simulink model "TBRe18_ECU_V7_AI"  (R2017b)
settings: Solver=FixedStepDiscrete  StartTime=0.0  StopTime=inf  FixedStep=0.0001  RelTol=1e-3
PostLoadFcn:
  | model_init();
libraries: simulink x16, simulink_extras x1
(part 4 of 4)

== system TBRe18_ECU_V7_AI/Data_Processing/Diagnostics/ECU_I//0s_Diagnostics/LV_Battery ==
  In1 : Inport
  Bus Creator : BusCreator  Inputs=3
  Bus Selector : BusSelector  OutputSignals=LV_Battery_Voltage
  Data Type Conversion : DataTypeConversion  OutDataTypeStr=uint8
  LV_Warning_% : simulink/Logic and Bit Operations/Compare To Constant  relop=<=  const=20  OutDataTypeStr=boolean
  Voltage_Act : Lookup_n-D  NumberOfTableDimensions=1  BreakpointsForDimension1=[0,20000]  Table=[500,33000]  TableDataTypeStr=Inherit: Inherit from 'Table data'  ExtrapMethod=Clip  UseLastTableValue=on  InternalRulePriority=Speed  RndMeth=Simplest  InputSameDT=on
  "Voltage_SOC " : Lookup_n-D  NumberOfTableDimensions=1  BreakpointsForDimension1=[1600, 24000, 25800, 26000, 26400]  Table=[0, 10, 20, 50, 100]  TableDataTypeStr=Inherit: Inherit from 'Table data'  ExtrapMethod=Clip  UseLastTableValue=on  InternalRulePriority=Speed  RndMeth=Simplest  InputSameDT=on
  Out1 : Outport
  wires:
  Bus Creator/1 -> Out1/1
  In1/1 -> Bus Selector/1
  LV_Warning_%/1 -> Bus Creator/1  "LV_Battery_Warning"
  "Voltage_SOC "/1 -> Data Type Conversion/1, LV_Warning_%/1
  Data Type Conversion/1 -> Bus Creator/2  "LV_Battery_SOC"
  Bus Selector/1 -> Voltage_Act/1, "Voltage_SOC "/1  "<LV_Battery_Voltage>"
  Voltage_Act/1 -> Bus Creator/3  "LV_Battery_Voltage"

== system TBRe18_ECU_V7_AI/Data_Processing/Diagnostics/ECU_I//0s_Diagnostics/Pedal_Box ==
  In1 : Inport
  APPS and BP Plausibility : MATLAB Function  TreatAsAtomicUnit=on
  APPS_Implausibility_Check : MATLAB Function  TreatAsAtomicUnit=on
  Bus Creator : BusCreator  Inputs=10
  Bus Selector : BusSelector  OutputSignals=Pedal_Box_Data.Throttle1_Voltage,Pedal_Box_Data.Throttle2_Voltage,Pedal_Box_Data.Brake_Voltage
  Ground : Ground
  Sensor_Diag : MATLAB Function  TreatAsAtomicUnit=on
  Terminator : Terminator
  Voltage_to_% Conversion : Subsystem
  prv_BSPD : Delay  DelayLength=1  InitialCondition=0
  Out1 : Outport
  wires:
  Bus Creator/1 -> Out1/1
  In1/1 -> Bus Selector/1
  Bus Selector/1 -> Sensor_Diag/1(TV_1), Bus Creator/1  "<Throttle1_Voltage>"
  Bus Selector/3 -> Sensor_Diag/3(BV_1), Bus Creator/3  "<Brake_Voltage>"
  APPS and BP Plausibility/2(APPS_BP_Implausibility) -> prv_BSPD/1, Bus Creator/10  "APPS_BP_Implausibility"
  APPS and BP Plausibility/1(Throttle_Percentage) -> Bus Creator/9  "Throttle_%"
  Sensor_Diag/1(Pedal_Sensor_Fail) -> APPS_Implausibility_Check/1(Pedal_Sensor_Fail), Bus Creator/4  "Pedal_Sensor_Fail"
  APPS_Implausibility_Check/1(APPS_Implausbility) -> Bus Creator/8  "APPS_Implausibility"
  APPS_Implausibility_Check/2(Throttle_Percentage) -> Terminator/1
  Voltage_to_% Conversion/3(Out3) -> APPS and BP Plausibility/2(Brake_In), Bus Creator/7
  Sensor_Diag/2(TV1_Out) -> Voltage_to_% Conversion/1(In1)
  Sensor_Diag/3(TV2_Out) -> Voltage_to_% Conversion/2(In2)
  Sensor_Diag/4(BV_Out) -> Voltage_to_% Conversion/3(In3)
  Voltage_to_% Conversion/1(Out1) -> APPS and BP Plausibility/1(Throttle_In), Bus Creator/5
  Bus Selector/2 -> Sensor_Diag/2(TV_2), Bus Creator/2  "<Throttle2_Voltage>"
  Voltage_to_% Conversion/2(Out2) -> Bus Creator/6, APPS_Implausibility_Check/3(Throttle2_Per)
  prv_BSPD/1 -> APPS and BP Plausibility/3(APPS_BP_Implausibility_Prv)
  Ground/1 -> APPS_Implausibility_Check/2(Throttle1_Per)

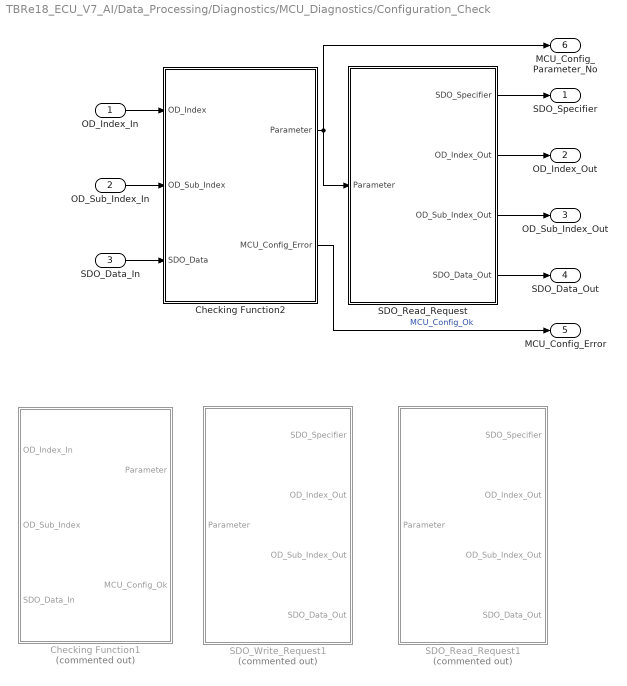
== system TBRe18_ECU_V7_AI/Data_Processing/Diagnostics/MCU_Diagnostics/Configuration_Check ==
  OD_Index_In : Inport
  OD_Sub_Index_In : Inport  Port=2
  SDO_Data_In : Inport  Port=3
  Checking Function1 : MATLAB Function  Commented=on  TreatAsAtomicUnit=on
  Checking Function2 : MATLAB Function  TreatAsAtomicUnit=on
  SDO_Read_Request : MATLAB Function  TreatAsAtomicUnit=on
  SDO_Read_Request1 : MATLAB Function  Commented=on  TreatAsAtomicUnit=on
  SDO_Write_Request1 : MATLAB Function  Commented=on  TreatAsAtomicUnit=on
  SDO_Specifier : Outport
  OD_Index_Out : Outport  Port=2
  OD_Sub_Index_Out : Outport  Port=3
  SDO_Data_Out : Outport  Port=4
  MCU_Config_Error : Outport  Port=5
  MCU_Config_Parameter_No : Outport  Port=6
  wires:
  Checking Function2/2(MCU_Config_Error) -> MCU_Config_Error/1  "MCU_Config_Ok"
  Checking Function2/1(Parameter) -> SDO_Read_Request/1(Parameter), MCU_Config_Parameter_No/1
  OD_Index_In/1 -> Checking Function2/1(OD_Index)
  SDO_Read_Request/3(OD_Sub_Index_Out) -> OD_Sub_Index_Out/1
  SDO_Data_In/1 -> Checking Function2/3(SDO_Data)
  SDO_Read_Request/1(SDO_Specifier) -> SDO_Specifier/1
  OD_Sub_Index_In/1 -> Checking Function2/2(OD_Sub_Index)
  SDO_Read_Request/4(SDO_Data_Out) -> SDO_Data_Out/1
  SDO_Read_Request/2(OD_Index_Out) -> OD_Index_Out/1

== system TBRe18_ECU_V7_AI/Data_Processing/Diagnostics/MCU_Diagnostics/Power Monitoring ==
  MCU_Input_Power : Inport
  Voltage_In : Inport  Port=2
  Current_In : Inport  Port=3
  Compare To Constant : simulink/Logic and Bit Operations/Compare To Constant  relop=>=  const=80000  OutDataTypeStr=boolean
  Gain : Gain  Gain=1000
  MinMax : MinMax  Function=max  Inputs=2
  Product : Product
  MCU_Power : Outport
  DC_Link_Voltage : Outport  Port=2
  DC_Link_Current : Outport  Port=3
  Power_Limit_Breach : Outport  Port=4
  wires:
  MinMax/1 -> Compare To Constant/1
  Voltage_In/1 -> Product/1, DC_Link_Voltage/1
  Current_In/1 -> Product/2, DC_Link_Current/1
  Product/1 -> MinMax/2
  Compare To Constant/1 -> Power_Limit_Breach/1
  MCU_Input_Power/1 -> Gain/1, MCU_Power/1
  Gain/1 -> MinMax/1

== system TBRe18_ECU_V7_AI/Data_Processing/Diagnostics/MCU_Diagnostics/Temp_Check ==
  MCU_Temp : Inport
  Motor_Temp : Inport  Port=2
  Max_Temp : simulink/Logic and Bit Operations/Compare To Constant  relop=>=  const=50  OutDataTypeStr=boolean
  MinMax : MinMax  Function=max  Inputs=2
  Pump_Start_Temp : simulink/Logic and Bit Operations/Compare To Constant  relop=>=  const=30  OutDataTypeStr=boolean
  MCU_Temperature : Outport
  Motor_Temperature : Outport  Port=2
  MCU_Motor_Temp_Error : Outport  Port=3
  MCU_Pump_Req : Outport  Port=4
  wires:
  MCU_Temp/1 -> MinMax/1, MCU_Temperature/1  "MCU_Temp"
  Motor_Temp/1 -> Motor_Temperature/1, MinMax/2  "Motor_Temp"
  MinMax/1 -> Pump_Start_Temp/1, Max_Temp/1
  Max_Temp/1 -> MCU_Motor_Temp_Error/1  "MCU_Motor_Temp_Error"
  Pump_Start_Temp/1 -> MCU_Pump_Req/1

== system TBRe18_ECU_V7_AI/Data_Processing/Vehicle_Functionality/Hardwired_Output_Functions/BSPD ==
  In1 : Inport
  In3 : Inport  Port=2
  Compare To Constant1 : simulink/Logic and Bit Operations/Compare To Constant  relop=>=  const=2500  OutDataTypeStr=boolean
  Compare To Constant2 : simulink/Logic and Bit Operations/Compare To Constant  relop=>=  const=2500  OutDataTypeStr=boolean
  Ground : Ground
  Logical Operator : Logic  AllPortsSameDT=off  OutDataTypeStr=boolean
  S-R Flip-Flop : simulink_extras/Flip Flops/S-R Flip-Flop  initial_condition=0
  Terminator : Terminator
  Out1 : Outport
  wires:
  Compare To Constant1/1 -> Logical Operator/1
  Compare To Constant2/1 -> Logical Operator/2
  Logical Operator/1 -> S-R Flip-Flop/1
  S-R Flip-Flop/1 -> Out1/1
  In1/1 -> Compare To Constant1/1
  In3/1 -> Compare To Constant2/1
  Ground/1 -> S-R Flip-Flop/2
  S-R Flip-Flop/2 -> Terminator/1

== system TBRe18_ECU_V7_AI/Data_Processing/Vehicle_Functionality/Vehicle_Operation_Mode/System_Error ==
  note: Shutdown Sig Not Working, BSPD dissconected
  In : Inport
  Bus Selector1 : BusSelector  OutputSignals=Shutdown_Data.Shutdown_Error,ECU_IO_Data.Pedal_Box_Data.APPS_BP_Implausibility,ECU_IO_Data.Pedal_Box_Data.APPS_Implausibility
  Ground : Ground
  Ground1 : Ground
  Ground2 : Ground
  Logical Operator : Logic  Operator=OR  Inputs=4  AllPortsSameDT=off  OutDataTypeStr=boolean
  Terminator : Terminator
  Terminator1 : Terminator
  Out : Outport
  wires:
  In/1 -> Bus Selector1/1  "Input_Data"
  Logical Operator/1 -> Out/1  "System_Error"
  Bus Selector1/1 -> Terminator/1  "<Shutdown_Error>"
  Bus Selector1/2 -> Terminator1/1  "<APPS_BP_Implausibility>"
  Bus Selector1/3 -> Logical Operator/4  "<APPS_Implausibility>"
  Ground/1 -> Logical Operator/1
  Ground1/1 -> Logical Operator/2
  Ground2/1 -> Logical Operator/3

== system TBRe18_ECU_V7_AI/Data_Processing/Diagnostics/ECU_I//0s_Diagnostics/Pedal_Box/Voltage_to_% Conversion ==
  In1 : Inport
  In2 : Inport  Port=2
  In3 : Inport  Port=3
  Data Type Conversion : DataTypeConversion  OutDataTypeStr=uint8
  Data Type Conversion1 : DataTypeConversion  OutDataTypeStr=uint8
  Data Type Conversion2 : DataTypeConversion  OutDataTypeStr=uint8
  Map1 : Lookup_n-D  NumberOfTableDimensions=1  BreakpointsForDimension1=[5170,6500]  Table=[0,100]  ExtrapMethod=Clip  UseLastTableValue=on  InternalRulePriority=Speed  RndMeth=Simplest  InputSameDT=on
  Map2 : Lookup_n-D  NumberOfTableDimensions=1  BreakpointsForDimension1=[6500,8000]  Table=[0,100]  ExtrapMethod=Clip  UseLastTableValue=on  InternalRulePriority=Speed  RndMeth=Simplest  InputSameDT=on
  Map3 : Lookup_n-D  NumberOfTableDimensions=1  BreakpointsForDimension1=[1300,5600]  Table=[0,100]  ExtrapMethod=Clip  UseLastTableValue=on  InternalRulePriority=Speed  RndMeth=Simplest  InputSameDT=on
  Out1 : Outport
  Out2 : Outport  Port=2
  Out3 : Outport  Port=3
  wires:
  Data Type Conversion/1 -> Out3/1  "Brake_%"
  In3/1 -> Map3/1
  In1/1 -> Map1/1
  In2/1 -> Map2/1
  Map3/1 -> Data Type Conversion/1
  Data Type Conversion1/1 -> Out1/1  "Throttle1_%"
  Map1/1 -> Data Type Conversion1/1
  Data Type Conversion2/1 -> Out2/1  "Throttle2_%"
  Map2/1 -> Data Type Conversion2/1

== matlab function TBRe18_ECU_V7_AI/Data_Processing/Vehicle_Functionality/Vehicle_Operation_Mode/Vehical Mode Selection ==
  data: Throttle input; Brake input; Reset input; Push_to_Start input; Error input; Prev_Operation_Mode input; MCU_NMT_Mode output; PWM output; Operation_Mode output; Buzzer output; Buzzer_Timer_In input; Buzzer_Timer_Out output; Precharge_Hold input
function [ MCU_NMT_Mode, PWM, Operation_Mode, Buzzer, Buzzer_Timer_Out] = Vehicle_Operation_Mode(Throttle, Brake,Reset, Push_to_Start,Error, Prev_Operation_Mode, Buzzer_Timer_In, Precharge_Hold)

%Parameter Initialisation
PWM = false;
Buzzer = false;
Buzzer_Timer_Out = 0;
Operation_Mode = Prev_Operation_Mode;

%Error checker
if (Error)
    Operation_Mode = uint8(0);
    MCU_NMT_Mode = uint8(0); %Stopped
end

%% -------------Vehicle Operation Modes--------------------%%

switch Operation_Mode
    
    case 0 %Error_Mode/No_Mode
        PWM = false;
        MCU_NMT_Mode = uint8(0); %Stopped Mode
        
        if (~Error)
            Operation_Mode = uint8(1);
        end
        
    case 1 %Standby_Mode: When car is first turned on
        PWM = false;
        MCU_NMT_Mode = uint8(2); %Pre-Operational Mode
        if (Brake && Push_to_Start && ~Throttle && (Precharge_Hold == 1))
            Operation_Mode = uint8(2);
            Buzzer_Timer_Out = 15;
        else
            Operation_Mode = uint8(1);
        end
        
    case 2 %Ready_to_Drive_Buzzer_Mode: Buzzer sounds before drive
        Buzzer = true;
        MCU_NMT_Mode = uint8(2); %Pre-Operational Mode
        if (Buzzer_Timer_In == 0)
            Buzzer = false;
            Operation_Mode = uint8(3);
        else
        Buzzer_Timer_Out = Buzzer_Timer_In - 1;
        Operation_Mode = uint8(2);
        end
        
    case 3 %Ready_to_Drive_Mode
        PWM = true;
        MCU_NMT_Mode = uint8(3); %Operational Mode
        if (Reset || (Precharge_Hold ~= 1))
            Operation_Mode = uint8(4);
        end
        
    case 4 %Reset Mode
        PWM = false;
        MCU_NMT_Mode = uint8(0); %Stopped Mode
        if (Reset)
            Operation_Mode = uint8(4); %Reset Mode
        else 
            Operation_Mode = uint8(0); %No Mode/Error Mode
        end
        
    otherwise 
        PWM = false;
        MCU_NMT_Mode = uint8(0);
        Operation_Mode = uint8(0);
end

end

== matlab function TBRe18_ECU_V7_AI/High_Priority_CAN_TX/MATLAB Function ==
  data: MCU_NMT_Mode input; Stopped output; Reset output; Pre_Op output; Op output
    function [Stopped,Reset,Pre_Op, Op]  = fcn(MCU_NMT_Mode)

Stopped = false;
Reset = false;
Pre_Op = false;
Op = false;

switch MCU_NMT_Mode
    case 0 %Stopped
        Stopped = true;
    case 1 %Reset
        Reset = true;
    case 2 %Pre-Op
        Pre_Op = true;
    case 3 %Op
        Op = true;
   
end

== matlab function TBRe18_ECU_V7_AI/Data_Processing/Diagnostics/BMS_Diagnostics/MATLAB Function ==
  data: Pack_Voltage input; Pre_Charge_Hold output; MCU_Link_Voltage input
function Pre_Charge_Hold = fcn(Pack_Voltage, MCU_Link_Voltage)
%Pre-Charge line hold
MCU_Link_Voltage = double(MCU_Link_Voltage);

Threshold = 0.90*Pack_Voltage;
%Added Check for voltage above 60V so precharge is not open when car turns
%on or no accumilator in car

if(((MCU_Link_Voltage/10) >= Threshold) && (MCU_Link_Voltage >= 60) && Pack_Voltage >= 200)
    Pre_Charge_Hold = true;
else
    Pre_Charge_Hold = false;
end

end

== matlab function TBRe18_ECU_V7_AI/Data_Processing/Diagnostics/MCU_Diagnostics/Configuration_Check/Checking Function1 ==
  data: Parameter output; OD_Index_In input; OD_Sub_Index input; SDO_Data_In input; MCU_Config_Ok output
function [Parameter, MCU_Config_Ok] = Checking(OD_Index_In,OD_Sub_Index, SDO_Data_In)
%Configuration parameter checking function
switch OD_Index_In
    case 0
        MCU_Config_Ok = false;
        Parameter = uint8(1);
        
    case 8244 %Motor type = 0 (PSM)
        MCU_Config_Ok = false;
        if (SDO_Data_In == 0)
            Parameter = uint8(2);
        else
            Parameter = uint8(1);
        end
        
    case 8249 %FOC_Delay = 1 (Enabled)
        if (SDO_Data_In == 1)
            MCU_Config_Ok = false;
            Parameter = uint8(3);
        else
            MCU_Config_Ok = false;
            Parameter = uint8(2);
        end
        
    case 8243 %Motor Pole Pairs = 10 Pole Pairs
        if (SDO_Data_In == 10)
            MCU_Config_Ok = false;
            Parameter = uint8(4);
        else
            MCU_Config_Ok = false;
            Parameter = uint8(3);
        end
        
    case 24693 %Motor Rated Current = 320A
        if (SDO_Data_In == 320000)
            MCU_Config_Ok = false;
            Parameter = uint8(5);
        else
            MCU_Config_Ok = false;
            Parameter = uint8(4);
        end
    case 24694 %Motor Rated Torque = 320Nm
        if (SDO_Data_In == 320000)
            MCU_Config_Ok = false;
            Parameter = uint8(6);
        else
            MCU_Config_Ok = false;
            Parameter = uint8(5);
        end
    case 8279 %Motor Temperature Sensor = 3 (kty 81/210)
        if (SDO_Data_In == 3)
            MCU_Config_Ok = false;
            Parameter = uint8(7);
        else
            MCU_Config_Ok = false;
            Parameter = uint8(6);
        end
        
        %%-----------FEEDBACK PARAMETERS-----------&&
    case 8256
        %Feedback Type
        if (SDO_Data_In == 2 && OD_Sub_Index == 1)
            MCU_Config_Ok = false;
            Parameter = uint8(8);
            
            %Feedback Resolution
        elseif (SDO_Data_In == 4096 && OD_Sub_Index == 6)
            MCU_Config_Ok = false;
            Parameter = uint8(9);
            
            %Auto aligning motor position current
        elseif (SDO_Data_In == 500 && OD_Sub_Index == 10)
            MCU_Config_Ok = false;
            Parameter = uint8(10);
            
            %Motor phase offset compensation
        elseif (SDO_Data_In == 190 && OD_Sub_Index == 8)
            MCU_Config_Ok = false;
            Parameter = uint8(11);
        else
            MCU_Config_Ok = false;
            Parameter = uint8(8);
        end
        
        %%-----------BATTERY PARAMETERS-----------&&
    case 8276 %Overvoltage limit = 400V
        if (SDO_Data_In == 400)
            MCU_Config_Ok = false;
            Parameter = uint8(12);
        else
            MCU_Config_Ok = false;
            Parameter = uint8(11);
        end
    case 8277
        %Undervoltage limit = 200V
        if (SDO_Data_In == 200 && OD_Sub_Index == 1)
            MCU_Config_Ok = false;
            Parameter = uint8(13);
            %Undervoltage limit gain = 20%/V
        elseif (SDO_Data_In == 20 && OD_Sub_Index == 2)
            MCU_Config_Ok = false;
            Parameter = uint8(14);
            %Undervoltage min voltage = 195V
        elseif (SDO_Data_In == 195 && OD_Sub_Index == 3)
            MCU_Config_Ok = false;
            Parameter = uint8(15);
        else
            MCU_Config_Ok = false;
            Parameter = uint8(12);
        end
        
    case 4112 %Parameter Save
        if (SDO_Data_In == 1702257011)
            MCU_Config_Ok = true;
            Parameter = uint8(0);
        else
            MCU_Config_Ok = false;
            Parameter = uint8(15);
        end
        
    otherwise
        MCU_Config_Ok = false;
        Parameter = uint8(1);
        
end
end

== matlab function TBRe18_ECU_V7_AI/Data_Processing/Diagnostics/MCU_Diagnostics/Configuration_Check/SDO_Write_Request1 ==
  data: Parameter input; SDO_Specifier output; OD_Index_Out output; OD_Sub_Index_Out output; SDO_Data_Out output
function [SDO_Specifier, OD_Index_Out, OD_Sub_Index_Out, SDO_Data_Out] = SDO_Write_Request(Parameter)
%Auto-align procedure parameter check

switch Parameter
    %%-----------MOTOR PARAMETERS-----------&&
    case 1 %Motor type
        SDO_Specifier = uint8(47); %Write
        OD_Index_Out = uint16(8244); %OD Index
        OD_Sub_Index_Out = uint8(0); %OD Sub-Index
        SDO_Data_Out = uint32(0); %SDO Data - specific value
    case 2 %FOC_Delay
        SDO_Specifier = uint8(47); %Write
        OD_Index_Out = uint16(8249); %OD Index
        OD_Sub_Index_Out = uint8(0); %OD Sub-Index
        SDO_Data_Out = uint32(1); %SDO Data - specific value
    case 3 %Motor Pole Pairs
        SDO_Specifier = uint8(47); %Write
        OD_Index_Out = uint16(8243); %OD Index
        OD_Sub_Index_Out = uint8(0); %OD Sub-Index
        SDO_Data_Out = uint32(10); %SDO Data - specific value
    case 4 %Motor Rated Current
        SDO_Specifier = uint8(47); %Write
        OD_Index_Out = uint16(24693); %OD Index
        OD_Sub_Index_Out = uint8(0); %OD Sub-Index
        SDO_Data_Out = uint32(320000); %SDO Data - specific value
    case 5 %Motor Rated Torque
        SDO_Specifier = uint8(47); %Write
        OD_Index_Out = uint16(24694); %OD Index
        OD_Sub_Index_Out = uint8(0); %OD Sub-Index
        SDO_Data_Out = uint32(320000); %SDO Data - specific value
    case 6 %Motor Temperature Sensor
        SDO_Specifier = uint8(47); %Write
        OD_Index_Out = uint16(8279); %OD Index
        OD_Sub_Index_Out = uint8(2); %OD Sub-Index
        SDO_Data_Out = uint32(3); %SDO Data - specific value
        
       %%-----------FEEDBACK PARAMETERS-----------&&
    case 7 %Feedback Type
        SDO_Specifier = uint8(47); %Write
        OD_Index_Out = uint16(8256); %OD Index
        OD_Sub_Index_Out = uint8(1); %OD Sub-Index
        SDO_Data_Out = uint32(2); %SDO Data - specific value
    case 8 %Feedback Resolution
        SDO_Specifier = uint8(47); %Write
        OD_Index_Out = uint16(8256); %OD Index
        OD_Sub_Index_Out = uint8(6); %OD Sub-Index
        SDO_Data_Out = uint32(4096); %SDO Data - specific value
    case 9 %Auto aligning motor position current
        SDO_Specifier = uint8(47); %Write
        OD_Index_Out = uint16(8256); %OD Index
        OD_Sub_Index_Out = uint8(10); %OD Sub-Index
        SDO_Data_Out = uint32(500); %SDO Data - specific value
    case 10 %Motor phase offset compensation
        SDO_Specifier = uint8(47); %Write
        OD_Index_Out = uint16(8256); %OD Index
        OD_Sub_Index_Out = uint8(8); %OD Sub-Index
        SDO_Data_Out = uint32(190); %SDO Data - specific value
        
        %%-----------BATTERY PARAMETERS-----------&&
    case 11 %Overvoltage limit
        SDO_Specifier = uint8(47); %Write
        OD_Index_Out = uint16(8276); %OD Index
        OD_Sub_Index_Out = uint8(1); %OD Sub-Index
        SDO_Data_Out = uint32(400); %SDO Data - specific value
    case 12 %Undervoltage limit
        SDO_Specifier = uint8(47); %Write
        OD_Index_Out = uint16(8277); %OD Index
        OD_Sub_Index_Out = uint8(1); %OD Sub-Index
        SDO_Data_Out = uint32(200); %SDO Data - specific value
    case 13 %Undervoltage limit gain
        SDO_Specifier = uint8(47); %Write
        OD_Index_Out = uint16(8277); %OD Index
        OD_Sub_Index_Out = uint8(2); %OD Sub-Index
        SDO_Data_Out = uint32(20); %SDO Data - specific value
    case 14 %Undervoltage min voltage
        SDO_Specifier = uint8(47); %Write
        OD_Index_Out = uint16(8277); %OD Index
        OD_Sub_Index_Out = uint8(3); %OD Sub-Index
        SDO_Data_Out = uint32(195); %SDO Data - specific value
    case 15 %Parameter Save
        SDO_Specifier = uint8(47); %Write
        OD_Index_Out = uint16(4112); %OD Index
        OD_Sub_Index_Out = uint8(1); %OD Sub-Index
        SDO_Data_Out = uint32(1702257011); %SDO Data - specific value
    otherwise
        SDO_Specifier = uint8(0); %Read
        OD_Index_Out = uint16(0); %OD Index
        OD_Sub_Index_Out = uint8(0); %OD Sub-Index
        SDO_Data_Out = uint32(0); %SDO Data - specific value
end

end

== matlab function TBRe18_ECU_V7_AI/Data_Processing/Diagnostics/MCU_Diagnostics/Configuration_Check/SDO_Read_Request ==
  data: Parameter input; SDO_Specifier output; OD_Index_Out output; OD_Sub_Index_Out output; SDO_Data_Out output
function [SDO_Specifier, OD_Index_Out, OD_Sub_Index_Out, SDO_Data_Out] = SDO_Read_Request(Parameter)
%Configuration procedure parameter check

switch Parameter
    %%-----------MOTOR PARAMETERS-----------&&
    case 1 %Motor type
        SDO_Specifier = uint8(64); %Read Request
        OD_Index_Out = uint16(8244); %OD Index
        OD_Sub_Index_Out = uint8(0); %OD Sub-Index
        SDO_Data_Out = uint32(0); %SDO Data - specific value
    case 2 %FOC_Delay
        SDO_Specifier = uint8(64); %Read Request
        OD_Index_Out = uint16(8249); %OD Index
        OD_Sub_Index_Out = uint8(0); %OD Sub-Index
        SDO_Data_Out = uint32(0); %SDO Data - specific value
    case 3 %Motor Pole Pairs
        SDO_Specifier = uint8(64); %Read Request
        OD_Index_Out = uint16(8243); %OD Index
        OD_Sub_Index_Out = uint8(0); %OD Sub-Index
        SDO_Data_Out = uint32(0); %SDO Data - specific value
    case 4 %Motor Rated Current
        SDO_Specifier = uint8(64); %Read Request
        OD_Index_Out = uint16(24693); %OD Index
        OD_Sub_Index_Out = uint8(0); %OD Sub-Index
        SDO_Data_Out = uint32(0); %SDO Data - specific value
    case 5 %Motor Rated Torque
        SDO_Specifier = uint8(64); %Read Request
        OD_Index_Out = uint16(24694); %OD Index
        OD_Sub_Index_Out = uint8(0); %OD Sub-Index
        SDO_Data_Out = uint32(0); %SDO Data - specific value
    case 6 %Motor Temperature Sensor
        SDO_Specifier = uint8(64); %Read Request
        OD_Index_Out = uint16(8279); %OD Index
        OD_Sub_Index_Out = uint8(1); %OD Sub-Index
        SDO_Data_Out = uint32(0); %SDO Data - specific value
        
       %%-----------FEEDBACK PARAMETERS-----------%%
    case 7 %Feedback Type
        SDO_Specifier = uint8(64); %Read Request
        OD_Index_Out = uint16(8256); %OD Index
        OD_Sub_Index_Out = uint8(1); %OD Sub-Index
        SDO_Data_Out = uint32(0); %SDO Data - specific value
    case 8 %Feedback Resolution
        SDO_Specifier = uint8(64); %Read Request
        OD_Index_Out = uint16(8256); %OD Index
        OD_Sub_Index_Out = uint8(6); %OD Sub-Index
        SDO_Data_Out = uint32(0); %SDO Data - specific value
    case 9 %Auto aligning motor position current
        SDO_Specifier = uint8(64); %Read Request
        OD_Index_Out = uint16(8256); %OD Index
        OD_Sub_Index_Out = uint8(10); %OD Sub-Index
        SDO_Data_Out = uint32(0); %SDO Data - specific value
    case 10 %Motor phase offset compensation
        SDO_Specifier = uint8(64); %Read Request
        OD_Index_Out = uint16(8256); %OD Index
        OD_Sub_Index_Out = uint8(8); %OD Sub-Index
        SDO_Data_Out = uint32(0); %SDO Data - specific value
        
        %%-----------BATTERY PARAMETERS-----------&&
    case 11 %Overvoltage limit
        SDO_Specifier = uint8(64); %Read Request
        OD_Index_Out = uint16(8276); %OD Index
        OD_Sub_Index_Out = uint8(0); %OD Sub-Index
        SDO_Data_Out = uint32(0); %SDO Data - specific value
    case 12 %Undervoltage limit
        SDO_Specifier = uint8(64); %Read Request
        OD_Index_Out = uint16(8277); %OD Index
        OD_Sub_Index_Out = uint8(1); %OD Sub-Index
        SDO_Data_Out = uint32(0); %SDO Data - specific value
    case 13 %Undervoltage limit gain
        SDO_Specifier = uint8(64); %Read Request
        OD_Index_Out = uint16(8277); %OD Index
        OD_Sub_Index_Out = uint8(2); %OD Sub-Index
        SDO_Data_Out = uint32(0); %SDO Data - specific value
    case 14 %Undervoltage min voltage
        SDO_Specifier = uint8(64); %Read Request
        OD_Index_Out = uint16(8277); %OD Index
        OD_Sub_Index_Out = uint8(3); %OD Sub-Index
        SDO_Data_Out = uint32(0); %SDO Data - specific value
    case 15 %Parameter Save
        SDO_Specifier = uint8(35); %Save
        OD_Index_Out = uint16(4112); %OD Index
        OD_Sub_Index_Out = uint8(1); %OD Sub-Index
        SDO_Data_Out = uint32(1702257011); %SDO Data - specific value
    otherwise
        SDO_Specifier = uint8(0); %Read
        OD_Index_Out = uint16(0); %OD Index
        OD_Sub_Index_Out = uint8(0); %OD Sub-Index
        SDO_Data_Out = uint32(0); %SDO Data - specific value
end

end

== matlab function TBRe18_ECU_V7_AI/Data_Processing/Diagnostics/MCU_Diagnostics/Configuration_Check/Checking Function2 ==
  data: Parameter output; OD_Index input; OD_Sub_Index input; SDO_Data input; MCU_Config_Error output
function [Parameter, MCU_Config_Error] = Checking(OD_Index,OD_Sub_Index, SDO_Data)
%Configuration parameter checking function
switch OD_Index
    case 0
        MCU_Config_Error = true;
        Parameter = uint8(1);
        
    case 8244 %Motor type = 0 (PSM)
        MCU_Config_Error = true;
        if (SDO_Data == 0)
            Parameter = uint8(2);
        else
            Parameter = uint8(1);
        end
        
    case 8249 %FOC_Delay = 1 (Enabled)
        if (SDO_Data == 1)
            MCU_Config_Error = true;
            Parameter = uint8(3);
        else
            MCU_Config_Error = true;
            Parameter = uint8(2);
        end
        
    case 8243 %Motor Pole Pairs = 10 Pole Pairs
        if (SDO_Data == 10)
            MCU_Config_Error = true;
            Parameter = uint8(4);
        else
            MCU_Config_Error = true;
            Parameter = uint8(3);
        end
        
    case 24693 %Motor Rated Current = 320A
        if (SDO_Data == 320000)
            MCU_Config_Error = true;
            Parameter = uint8(5);
        else
            MCU_Config_Error = true;
            Parameter = uint8(4);
        end
    case 24694 %Motor Rated Torque = 320Nm
        if (SDO_Data == 320000)
            MCU_Config_Error = true;
            Parameter = uint8(6);
        else
            MCU_Config_Error = true;
            Parameter = uint8(5);
        end
    case 8279 %Motor Temperature Sensor = 3 (kty 81/210)
        if (SDO_Data == 3)
            MCU_Config_Error = true;
            Parameter = uint8(7);
        else
            MCU_Config_Error = true;
            Parameter = uint8(6);
        end
        
        %%-----------FEEDBACK PARAMETERS-----------&&
    case 8256
        %Feedback Type
        if (SDO_Data == 2 && OD_Sub_Index == 1)
            MCU_Config_Error = true;
            Parameter = uint8(8);
            
            %Feedback Resolution
        elseif (SDO_Data == 4096 && OD_Sub_Index == 6)
            MCU_Config_Error = true;
            Parameter = uint8(9);
            
            %Auto aligning motor position current
        elseif (SDO_Data == 500 && OD_Sub_Index == 10)
            MCU_Config_Error = true;
            Parameter = uint8(10);
            
            %Motor phase offset compensation
        elseif (SDO_Data == 190 && OD_Sub_Index == 8)
            MCU_Config_Error = true;
            Parameter = uint8(11);
        else
            MCU_Config_Error = true;
            Parameter = uint8(7);
        end
        
        %%-----------BATTERY PARAMETERS-----------&&
    case 8276 %Overvoltage limit = 400V
        if (SDO_Data == 400)
            MCU_Config_Error = true;
            Parameter = uint8(12);
        else
            MCU_Config_Error = true;
            Parameter = uint8(11);
        end
    case 8277
        %Undervoltage limit = 200V
        if (SDO_Data == 200 && OD_Sub_Index == 1)
            MCU_Config_Error = true;
            Parameter = uint8(13);
            %Undervoltage limit gain = 20%/V
        elseif (SDO_Data == 20 && OD_Sub_Index == 2)
            MCU_Config_Error = true;
            Parameter = uint8(14);
            %Undervoltage min voltage = 195V
        elseif (SDO_Data == 195 && OD_Sub_Index == 3)
            MCU_Config_Error = true;
            Parameter = uint8(15);
        else
            MCU_Config_Error = true;
            Parameter = uint8(12);
        end
    case 4112 %Save Parameter
        MCU_Config_Error = false;
        Parameter = uint8(0);
        
    otherwise
        MCU_Config_Error = true;
        Parameter = uint8(1);
        
end
end

== matlab function TBRe18_ECU_V7_AI/Data_Processing/Diagnostics/MCU_Diagnostics/Configuration_Check/SDO_Read_Request1 ==
  data: Parameter input; SDO_Specifier output; OD_Index_Out output; OD_Sub_Index_Out output; SDO_Data_Out output
function [SDO_Specifier, OD_Index_Out, OD_Sub_Index_Out, SDO_Data_Out] = SDO_Read_Request(Parameter)
%Auto-align procedure parameter check

switch Parameter
    %%-----------MOTOR PARAMETERS-----------&&
    case 1 %Motor type
        SDO_Specifier = uint8(64); %Read Request
        OD_Index_Out = uint16(8244); %OD Index
        OD_Sub_Index_Out = uint8(0); %OD Sub-Index
        SDO_Data_Out = uint32(0); %SDO Data - specific value
    case 2 %FOC_Delay
        SDO_Specifier = uint8(64); %Read Request
        OD_Index_Out = uint16(8249); %OD Index
        OD_Sub_Index_Out = uint8(0); %OD Sub-Index
        SDO_Data_Out = uint32(0); %SDO Data - specific value
    case 3 %Motor Pole Pairs
        SDO_Specifier = uint8(64); %Read Request
        OD_Index_Out = uint16(8243); %OD Index
        OD_Sub_Index_Out = uint8(0); %OD Sub-Index
        SDO_Data_Out = uint32(0); %SDO Data - specific value
    case 4 %Motor Rated Current
        SDO_Specifier = uint8(64); %Read Request
        OD_Index_Out = uint16(24693); %OD Index
        OD_Sub_Index_Out = uint8(0); %OD Sub-Index
        SDO_Data_Out = uint32(0); %SDO Data - specific value
    case 5 %Motor Rated Torque
        SDO_Specifier = uint8(64); %Read Request
        OD_Index_Out = uint16(24694); %OD Index
        OD_Sub_Index_Out = uint8(0); %OD Sub-Index
        SDO_Data_Out = uint32(0); %SDO Data - specific value
    case 6 %Motor Temperature Sensor
        SDO_Specifier = uint8(64); %Read Request
        OD_Index_Out = uint16(8279); %OD Index
        OD_Sub_Index_Out = uint8(1); %OD Sub-Index
        SDO_Data_Out = uint32(0); %SDO Data - specific value
        
       %%-----------FEEDBACK PARAMETERS-----------%%
    case 7 %Feedback Type
        SDO_Specifier = uint8(64); %Read Request
        OD_Index_Out = uint16(8256); %OD Index
        OD_Sub_Index_Out = uint8(1); %OD Sub-Index
        SDO_Data_Out = uint32(0); %SDO Data - specific value
    case 8 %Feedback Resolution
        SDO_Specifier = uint8(64); %Read Request
        OD_Index_Out = uint16(8256); %OD Index
        OD_Sub_Index_Out = uint8(6); %OD Sub-Index
        SDO_Data_Out = uint32(0); %SDO Data - specific value
    case 9 %Auto aligning motor position current
        SDO_Specifier = uint8(64); %Read Request
        OD_Index_Out = uint16(8256); %OD Index
        OD_Sub_Index_Out = uint8(10); %OD Sub-Index
        SDO_Data_Out = uint32(0); %SDO Data - specific value
    case 10 %Motor phase offset compensation
        SDO_Specifier = uint8(64); %Read Request
        OD_Index_Out = uint16(8256); %OD Index
        OD_Sub_Index_Out = uint8(8); %OD Sub-Index
        SDO_Data_Out = uint32(0); %SDO Data - specific value
        
        %%-----------BATTERY PARAMETERS-----------&&
    case 11 %Overvoltage limit
        SDO_Specifier = uint8(64); %Read Request
        OD_Index_Out = uint16(8276); %OD Index
        OD_Sub_Index_Out = uint8(0); %OD Sub-Index
        SDO_Data_Out = uint32(0); %SDO Data - specific value
    case 12 %Undervoltage limit
        SDO_Specifier = uint8(64); %Read Request
        OD_Index_Out = uint16(8277); %OD Index
        OD_Sub_Index_Out = uint8(1); %OD Sub-Index
        SDO_Data_Out = uint32(0); %SDO Data - specific value
    case 13 %Undervoltage limit gain
        SDO_Specifier = uint8(64); %Read Request
        OD_Index_Out = uint16(8277); %OD Index
        OD_Sub_Index_Out = uint8(2); %OD Sub-Index
        SDO_Data_Out = uint32(0); %SDO Data - specific value
    case 14 %Undervoltage min voltage
        SDO_Specifier = uint8(64); %Read Request
        OD_Index_Out = uint16(8277); %OD Index
        OD_Sub_Index_Out = uint8(3); %OD Sub-Index
        SDO_Data_Out = uint32(0); %SDO Data - specific value
    case 15 %Parameter Save
        SDO_Specifier = uint8(35); %Save
        OD_Index_Out = uint16(4112); %OD Index
        OD_Sub_Index_Out = uint8(1); %OD Sub-Index
        SDO_Data_Out = uint32(1702257011); %SDO Data - specific value
    otherwise
        SDO_Specifier = uint8(0); %Read
        OD_Index_Out = uint16(0); %OD Index
        OD_Sub_Index_Out = uint8(0); %OD Sub-Index
        SDO_Data_Out = uint32(0); %SDO Data - specific value
end

end

== matlab function TBRe18_ECU_V7_AI/Data_Processing/Diagnostics/ECU_I//0s_Diagnostics/Pedal_Box/Sensor_Diag ==
  data: TV_1 input; Pedal_Sensor_Fail output; TV_2 input; TV1_Out output; TV2_Out output; BV_1 input; BV_Out output
function [Pedal_Sensor_Fail,TV1_Out,TV2_Out,BV_Out ] = Sensor_Diagnostics(TV_1,TV_2,BV_1)
%Checks whether the throttle sensors are in their calibrated range

%Initialisation of throttle outputs, default low 
TV1_Out=uint16(0);
TV2_Out=uint16(0);
BV_Out=uint16(0);

if (TV_1>8000 || TV_1<4000) %if V1 out of normal range
    Pedal_Sensor_Fail = uint8(1);
    if (TV_2>10000 || TV_2<6000)
        Pedal_Sensor_Fail = uint8(3); %if both throttle sensors out of normal range
    end
    if (BV_1>17000 || BV_1<0)
        Pedal_Sensor_Fail = uint8(5); %if all sensors out of normal range
    end
    
elseif (TV_2>10000 || TV_2<6000) %if V2 out of normal range
    Pedal_Sensor_Fail = uint8(2);
    
elseif (BV_1>17000 || BV_1<0) %if brake out of normal range
    Pedal_Sensor_Fail = uint8(4);

else %if no error pass voltages to pedal checks
    Pedal_Sensor_Fail= uint8(0);
    TV1_Out=uint16(TV_1);
    TV2_Out=uint16(TV_2);
    BV_Out=uint16(BV_1);
end

== matlab function TBRe18_ECU_V7_AI/Data_Processing/Diagnostics/ECU_I//0s_Diagnostics/Pedal_Box/APPS_Implausibility_Check ==
  data: Pedal_Sensor_Fail input; APPS_Implausbility output; Throttle1_Per input; Throttle2_Per input; Throttle_Percentage output
function [APPS_Implausbility, Throttle_Percentage] = APPS_Implausibility_Check(Pedal_Sensor_Fail, Throttle1_Per, Throttle2_Per)
%Limit generation for comparison
Upper_Limit = Throttle1_Per+15;
Lower_Limit = Throttle1_Per-15;

%Passes one throttle if in range and no pedal sensor errors
if ((Lower_Limit <= Throttle2_Per) && (Throttle2_Per <= Upper_Limit)&& Pedal_Sensor_Fail == 0)
    Throttle_Percentage = uint8(min(Throttle1_Per, Throttle2_Per));
    APPS_Implausbility = false;
%All other conditions result in no throttle being applied
else 
    Throttle_Percentage = uint8(0);
    APPS_Implausbility = true;
end 

end

== matlab function TBRe18_ECU_V7_AI/Data_Processing/Diagnostics/ECU_I//0s_Diagnostics/Pedal_Box/APPS and BP Plausibility ==
  data: Throttle_In input; Throttle_Percentage output; Brake_In input; APPS_BP_Implausibility output; APPS_BP_Implausibility_Prv input
function [Throttle_Percentage, APPS_BP_Implausibility] = APPS_BP_Plausibility_Check(Throttle_In, Brake_In, APPS_BP_Implausibility_Prv)
%Plausibility check on both throttle and brake

%Implausible case: when both brake and throttle applied
if (Brake_In >=20 && Throttle_In > 25)
    APPS_BP_Implausibility = true;
    Throttle_Percentage =uint8(0);
    
%Implausible case: when brake lifted but throttle still not below 5%
elseif (APPS_BP_Implausibility_Prv && Throttle_In > 5)
    APPS_BP_Implausibility = true;
    Throttle_Percentage =uint8(0);
    
%Plausible case, throttle goes below 5%
elseif (APPS_BP_Implausibility_Prv && Throttle_In < 5)
    APPS_BP_Implausibility = false;
    Throttle_Percentage =uint8(Throttle_In);
    
%Plausible case, normal operation
else
    APPS_BP_Implausibility = false;
    Throttle_Percentage =uint8(Throttle_In);
end

== matlab function TBRe18_ECU_V7_AI/Data_Processing/Vehicle_Functionality/Vehicle_Operation_Mode/Vehcile Mode No Reset ==
  data: Throttle input; Brake input; Push_to_Start input; Pre_Charge_Hold input; DriverlessRTD input; Error input; Prev_Operation_Mode input; Timer_In input; MCU_NMT_Mode output; PWM output; Operation_Mode output; Buzzer output; Timer_Out output
function [ MCU_NMT_Mode, PWM, Operation_Mode, Buzzer, Timer_Out] = Vehicle_Operation_Mode(Throttle, Brake, Push_to_Start, Pre_Charge_Hold, DriverlessRTD, Error, Prev_Operation_Mode, Timer_In)

%Parameter Initialisation
PWM = false;
Buzzer = false;
Timer_Out = uint8(0);
Operation_Mode = Prev_Operation_Mode;

%Error checker
if (Error)
    Operation_Mode = uint8(0);
    MCU_NMT_Mode = uint8(0); %Stopped
end

%% -------------Vehicle Operation Modes--------------------%%

switch Operation_Mode
    
    case 0 %Error_Mode/No_Mode
        PWM = false;
        MCU_NMT_Mode = uint8(0); %Stopped Mode
        
        if (~Error)
            Operation_Mode = uint8(1);
        end
        
    case 1 %Standby_Mode: When car is first turned on
        PWM = false;
        MCU_NMT_Mode = uint8(2); %Pre-Operational Mode
        if ((Brake && Push_to_Start && ~Throttle && Pre_Charge_Hold)||(Brake && DriverlessRTD && ~Throttle && Pre_Charge_Hold))
            Operation_Mode = uint8(2);
            Timer_Out = uint8(30); %1.5s
        elseif (Push_to_Start)
            Operation_Mode = uint8(0);
        else
            Operation_Mode = uint8(1);
        end
        
    case 2 %Ready_to_Drive_Buzzer_Mode: Buzzer sounds before drive
        Buzzer = true;
        MCU_NMT_Mode = uint8(2); %Pre-Operational Mode
        if (Timer_In == uint8(0))
            Buzzer = false;
            Operation_Mode = uint8(3);
        else
            Timer_Out = Timer_In - uint8(1);
            Operation_Mode = uint8(2);
        end
        
    case 3 %Ready_to_Drive_Mode
        PWM = true;
        MCU_NMT_Mode = uint8(3); %Operational Mode
        
        if (Push_to_Start||~Pre_Charge_Hold||~DriverlessRTD)
            Operation_Mode = uint8(0);
        end
        
    otherwise
        PWM = false;
        MCU_NMT_Mode = uint8(0);
        Operation_Mode = uint8(0);
end

end

== stateflow chart TBRe18_ECU_V7_AI/Data_Processing/Vehicle_Functionality/Vehicle_Operation_Mode/Chart ==
  state Standby State:
    Buzzer = false;
    PWM = false;
    MCU_NMT_Mode = uint8(2); %Pre-Operational Mode
  state Error State:
    Buzzer = false;
    PWM = false;
    MCU_NMT_Mode = uint8(0); %Stopped Mode
  state Buzzer State:
    PWM = false;
    Buzzer = true;
    MCU_NMT_Mode = uint8(2); %Pre-Operational Mode
  state R2D State:
    Buzzer = false;
    PWM = true;
    MCU_NMT_Mode = uint8(3); %Operational Mode
  (default) -> Error State:
  Error State: -> Standby State: : [~Error]
  Standby State: -> Error State: [order 1] : [Error || (btnDash && ~Brake)]
  R2D State: -> Error State: : [Error || btnDaash]
  Buzzer State: -> Error State: [order 1] : [Error]
  Standby State: -> Buzzer State: [order 2] : [btnDash && Brake && ~Throttle]
  Buzzer State: -> R2D State: [order 2] : after(1.5,sec)
